simulink model "mod_semplificato"  (R2014a)
settings: Solver=ode45  StartTime=0.0  StopTime=50  RelTol=1e-3
libraries: cstblocks x2, simulink x1
settings Model: Creator=HP  LastModifiedBy=HP

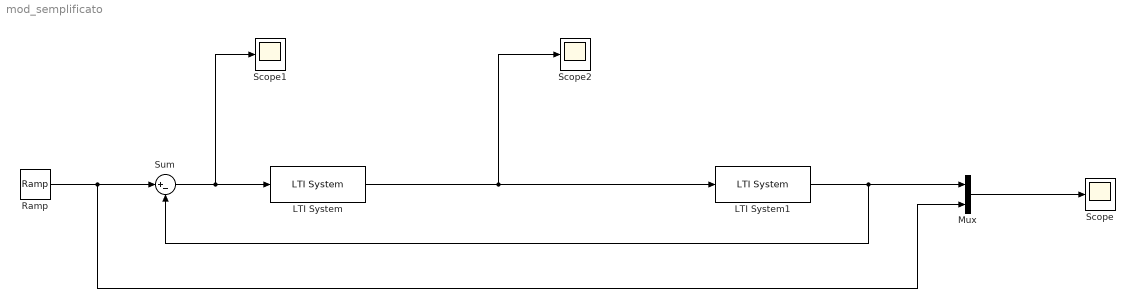
== system mod_semplificato ==
  LTI System : cstblocks/LTI System  sys=C_discreto  IC=[]
  LTI System1 : cstblocks/LTI System  sys=F_primo  IC=[]
  Mux : Mux  Inputs=2
  Ramp : simulink/Sources/Ramp  slope=1  start=0  X0=0
  Scope : Scope
  Scope1 : Scope
  Scope2 : Scope
      settings: SaveName=ScopeData2
  Sum : Sum  Inputs=|+-
  wires:
  Ramp/1 -> Mux/2, Sum/1
  Sum/1 -> Scope1/1, LTI System/1
  LTI System/1 -> Scope2/1, LTI System1/1
  LTI System1/1 -> Sum/2, Mux/1
  Mux/1 -> Scope/1
